simulink model "lin_with_Observer"  (R2019b)
settings: Solver=VariableStepAuto  StartTime=0.0  StopTime=10  RelTol=1e-3
undefined symbols (not defined in the file or in its folder): sigbuilder_block
libraries: mpclib x1, simulink x1, cstblocks x1
settings Model: Creator=gautamsharma  LastModifiedBy=chait

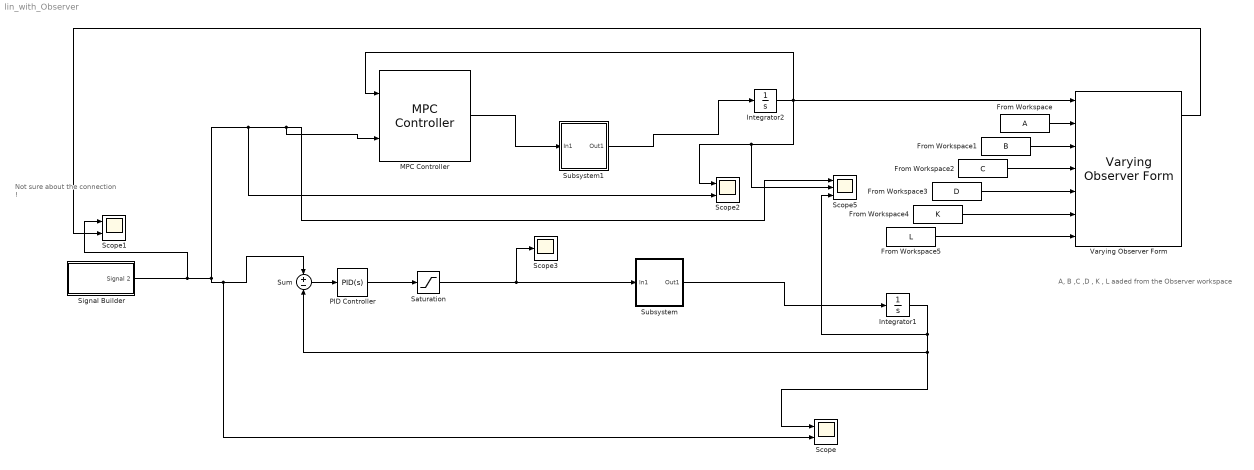
== system lin_with_Observer ==
  note: A, B ,C ,D , K , L aaded from the Observer workspace
  note: Not sure about the connection !
  From Workspace : FromWorkspace  VariableName=A  SampleTime=0
  From Workspace1 : FromWorkspace  VariableName=B  SampleTime=0
  From Workspace2 : FromWorkspace  VariableName=C  SampleTime=0
  From Workspace3 : FromWorkspace  VariableName=D  SampleTime=0
  From Workspace4 : FromWorkspace  VariableName=K  SampleTime=0
  From Workspace5 : FromWorkspace  VariableName=L  SampleTime=0
  Integrator1 : Integrator
  Integrator2 : Integrator
  MPC Controller : mpclib/MPC Controller  SCDEnableBlockLinearizationSpecification=on  mpcobj=mpc1  is_multiple=0  enable_value=0  return_u0=off  updateMPCinCallerWorkspace=on  md_inport=off  mv_inport=off  uref_inport=off  return_cost=off  return_mvseq=off  return_qpstatus=off  return_xseq=off  return_state=off  return_ovseq=off  state_inport=off  umin_inport=off  umax_inport=off  ymin_inport=off  ymax_inport=off  cc_inport=off  ywt_inport=off  uwt_inport=off  duwt_inport=off  rhoeps_inport=off  pm_inport=off  MaximumP=10  HorizonChoice=FixedHorizon  n_ts=0.01  n_p=10  n_mv=1  n_md=0  n_ud=0  n_mo=1  n_uo=0  BlockDataType=double  SampleTimeInherited=off  switch_inport=off
  PID Controller : simulink/Continuous/PID Controller  Controller=PID  Form=Parallel  TimeDomain=Continuous-time  SampleTime=-1  IntegratorMethod=Forward Euler  FilterMethod=Forward Euler  ControllerParametersSource=internal  P=0.0540540930744823  I=0.00396527995749108  D=0.0998499702123111  UseFilter=on  N=1142.8279760416  TunerSelectOption=Transfer Function Based (PID Tuner App)  InitialConditionSource=internal  InitialConditionForIntegrator=0  InitialConditionForFilter=0  DifferentiatorICPrevScaledInput=0  ExternalReset=none  TrackingMode=off  Kt=1  LimitOutput=off  UpperSaturationLimit=inf  LowerSaturationLimit=-inf  LinearizeAsGain=on  AntiWindupMode=none  Kb=1  POutMin=[]  POutMax=[]  IOutMin=[]  IOutMax=[]  DOutMin=[]  DOutMax=[]  NOutMin=[]  NOutMax=[]  SumOutMin=[]  SumOutMax=[]  SaturationOutMin=[]  SaturationOutMax=[]  PParamMin=[]  PParamMax=[]  IParamMin=[]  IParamMax=[]  DParamMin=[]  DParamMax=[]  NParamMin=[]  NParamMax=[]  KbParamMin=[]  KbParamMax=[]  KtParamMin=[]  KtParamMax=[]  KbOutMin=[]  KbOutMax=[]  KtOutMin=[]  KtOutMax=[]  IntegratorOutMin=[]  IntegratorOutMax=[]  FilterOutMin=[]  FilterOutMax=[]  SumI1OutMin=[]  SumI1OutMax=[]  SumI2OutMin=[]  SumI2OutMax=[]  SumI3OutMin=[]  SumI3OutMax=[]  SumI4OutMin=[]  SumI4OutMax=[]  SumDOutMin=[]  SumDOutMax=[]  DifferentiatorOutMin=[]  DifferentiatorOutMax=[]  FilterDiffOutCoefMin=[]  FilterDiffOutCoefMax=[]  ReciprocalOutMin=[]  ReciprocalOutMax=[]  SumDenOutMin=[]  SumDenOutMax=[]  SumNumOutMin=[]  SumNumOutMax=[]  DivideOutMin=[]  DivideOutMax=[]  IntegratorContinuousStateAttributes=''  IntegratorStateMustResolveToSignalObject=off  IntegratorRTWStateStorageClass=Auto  FilterContinuousStateAttributes=''  FilterStateMustResolveToSignalObject=off  FilterRTWStateStorageClass=Auto  ParallelPVariant=InternalParameters  IdealPVariant=Disabled  IVariant=InternalParameters  DVariant=InternalParameters  IntegratorVariant=Continuous  SatVariant=Disabled  AWVariant=Passthrough  PCopyVariant=Disabled  TRVariant=Disabled  FdbkBlocksVariant=Forward  IdealPFdbkVariant=Disabled  SatFdbkVariant=Disabled  DerivativeFilterVariant=ContFilter  NVariant=InternalParameters  NCopyVariant=Disabled  FilterICVariant=InternalICsFilter  IntegratorICVariant=InternalICs  ExternalResetVariant=Disabled  TRSumVariant=Passthrough  SumFdbkVariant=Disabled  SumVariant=Sum_PID
  Saturation : Saturate  UpperLimit=pi/6  LowerLimit=-pi/6
  Scope : Scope  NumInputPorts=2
  Scope1 : Scope  NumInputPorts=2
  Scope2 : Scope  NumInputPorts=2
  Scope3 : Scope
  Scope5 : Scope  NumInputPorts=3
  Signal Builder : Subsystem  Tag=STV Subsys  LoadFcn=sigbuilder_block('load');  StartFcn=sigbuilder_block('start');  StopFcn=sigbuilder_block('stop');  ClipboardFcn=sigbuilder_block('clipboard');  mask(Sigbuilder block){tuvar=[0:10]}
      mask help: Simulink:masks:SigbuilderBlock_MD
      mask init:
      | if ~strcmp(get_param(bdroot(gcbh),'SimulationStatus'),'stopped') tuvar = sigbuilder_block('maskInit'); end
      settings: CopyFcn=sigbuilder_block('copy');  DeleteFcn=sigbuilder_block('delete');  ModelCloseFcn=sigbuilder_block('modelClose');  PreSaveFcn=sigbuilder_block('preSave');  PauseFcn=sigbuilder_block('pause');  ContinueFcn=sigbuilder_block('continue');  NameChangeFcn=sigbuilder_block('namechange');  OpenFcn=sigbuilder_block('open',[0 45 1280 659 ]);  CloseFcn=sigbuilder_block('close');
      mask Display: plot(0, 0, 100, 100,[2, 2, 32, 32, 2], [68, 8, 8, 68, 68],[32, 2], [38, 38], [32, 19, 2],[53, 60, 44], [32, 17, 17, 2],[16, 16, 31, 31]);txt = getActiveGroup(gcbh);text(2, 100, txt,'verticalAlignment', 'top');
  Subsystem : Subsystem
  Subsystem1 : Subsystem
  Sum : Sum  Inputs=+-
  Varying Observer Form : cstblocks/Linear Parameter Varying/Varying Observer Form  x0=0  xNames=''  OutputX=on  OutputDX=on
      settings: SourceProductName=Control System Toolbox  SourceProductBaseCode=CT
  wires:
  Integrator1/1 -> Sum/2, Scope/1, Scope5/3
  Subsystem/1(Out1) -> Integrator1/1
  Subsystem1/1(Out1) -> Integrator2/1
  Integrator2/1 -> Scope5/2, Scope2/1, Varying Observer Form/1, MPC Controller/1
  Signal Builder/1(Signal 2) -> Scope1/1, MPC Controller/2, Scope5/1, Scope2/2, Scope/2, Sum/1
  Saturation/1 -> Scope3/1, Subsystem/1(In1)
  Sum/1 -> PID Controller/1
  PID Controller/1 -> Saturation/1
  MPC Controller/1 -> Subsystem1/1(In1)
  From Workspace2/1 -> Varying Observer Form/4
  From Workspace/1 -> Varying Observer Form/2
  From Workspace4/1 -> Varying Observer Form/6
  From Workspace3/1 -> Varying Observer Form/5
  From Workspace5/1 -> Varying Observer Form/7
  From Workspace1/1 -> Varying Observer Form/3
  Varying Observer Form/1 -> Scope1/2

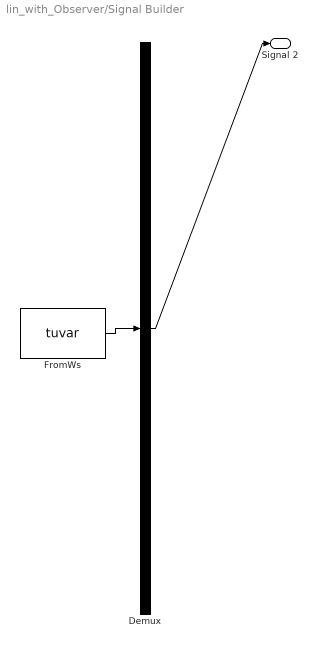
== system lin_with_Observer/Signal Builder ==
  Demux : Demux  Tag=STV Demux  Outputs=1
  FromWs : FromWorkspace  Tag=STV FromWs  VariableName=tuvar  SampleTime=0
      SigBuilderData=|
      | common.afterFinalStr = 'Extrapolate'
      | common.sampleTime = 0
      | dataSet.timeRange = [0 10]
      | dataSet.name = 'Group 1'
      | sbobj.Groups.Name = 'Group 1'
      | sbobj.Groups.Signals.Name = 'Signal 2'
      | sbobj.Groups.Signals.XData = [0 1 2 3 4 5 6 7 8 9 10]
      | sbobj.Groups.Signals.YData = [-0.3 0.06 0.8 1.7 2.8 3.54 4 4.06 4.04 4.06 4]
  Signal 2 : Outport  Tag=STV Outport
  wires:
  FromWs/1 -> Demux/1
  Demux/1 -> Signal 2/1

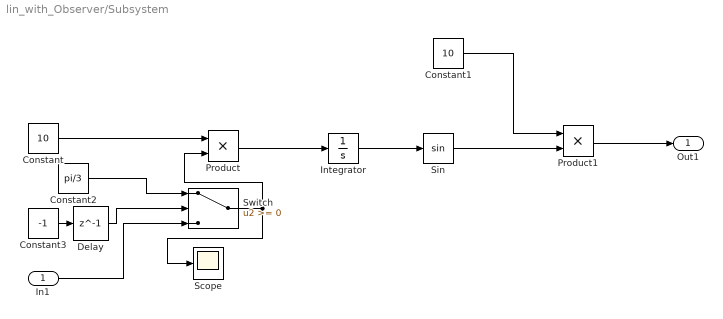
== system lin_with_Observer/Subsystem ==
  In1 : Inport
  Constant : Constant  Value=10
  Constant1 : Constant  Value=10
  Constant2 : Constant  Value=pi/3
  Constant3 : Constant  Value=-1
  Delay : Delay  DelayLength=1
  Integrator : Integrator
  Product : Product
  Product1 : Product
  Scope : Scope
  Sin : Trigonometry
  Switch : Switch
  Out1 : Outport
  wires:
  Product1/1 -> Out1/1
  Sin/1 -> Product1/2
  Constant1/1 -> Product1/1
  Integrator/1 -> Sin/1
  Product/1 -> Integrator/1
  Constant/1 -> Product/1
  Constant2/1 -> Switch/1
  In1/1 -> Switch/3
  Constant3/1 -> Delay/1
  Delay/1 -> Switch/2
  Switch/1 -> Product/2, Scope/1

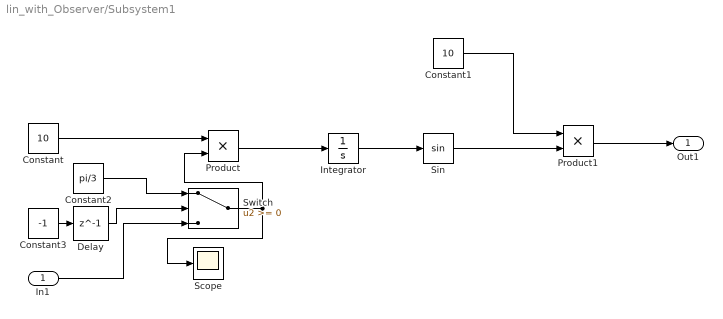
== system lin_with_Observer/Subsystem1 ==
  In1 : Inport
  Constant : Constant  Value=10
  Constant1 : Constant  Value=10
  Constant2 : Constant  Value=pi/3
  Constant3 : Constant  Value=-1
  Delay : Delay  DelayLength=1
  Integrator : Integrator
  Product : Product
  Product1 : Product
  Scope : Scope
  Sin : Trigonometry
  Switch : Switch
  Out1 : Outport
  wires:
  Switch/1 -> Scope/1, Product/2
  Delay/1 -> Switch/2
  Constant3/1 -> Delay/1
  In1/1 -> Switch/3
  Constant2/1 -> Switch/1
  Constant/1 -> Product/1
  Product/1 -> Integrator/1
  Integrator/1 -> Sin/1
  Constant1/1 -> Product1/1
  Sin/1 -> Product1/2
  Product1/1 -> Out1/1
